simulink model "myGuyton_corrected_new"  (Simulink 6.6)
settings: Solver=ode15s  StartTime=0  StopTime=60*24*14  FixedStep=0.025  MaxStep=1  MinStep=0.00000001  RelTol=1e-1
values from neighbouring files (symbols this model uses):
  A1K = 0.5    [G92_var_decl_exp.m]
  A2K = 60    [G92_var_decl_exp.m]
  A3K = 40000    [G92_var_decl_exp.m]
  A4K = 0.1    [G92_var_decl_exp.m]
  A4K2 = 40000    [G92_var_decl_exp.m]
  AARK = 1    [G92_var_decl_exp.m]
  AARLL = 4    [G92_var_decl_exp.m]
  ADHC_IC = 1.01449    [G92_var_decl_exp.m]
  ADHINF = 0    [G92_var_decl_exp.m]
  ADHKLL = 0.2    [G92_var_decl_exp.m]
  ADHKUL = 5    [G92_var_decl_exp.m]
  ADHPAM = 0.3    [G92_var_decl_exp.m]
  ADHPUL = 85    [G92_var_decl_exp.m]
  ADHTC = 15    [G92_var_decl_exp.m]
  ADHVLL = 0.93617    [G92_var_decl_exp.m]
  ADHVUL = 2.5    [G92_var_decl_exp.m]
  AH10 = 0.333    [G92_var_decl_exp.m]
  AH11 = 1000    [G92_var_decl_exp.m]
  AH9 = 1    [G92_var_decl_exp.m]
  AHMNAR = 0.3    [G92_var_decl_exp.m]
  AHTHM = 2    [G92_var_decl_exp.m]
  AHY_IC = -0.461862    [G92_var_decl_exp.m]
  ALCLK = 0.3    [G92_var_decl_exp.m]
  ALDINF = 0    [G92_var_decl_exp.m]
  ALDKNS = 0    [G92_var_decl_exp.m]
  ALDMM = 2.5    [G92_var_decl_exp.m]
  AM1LL = 0    [G92_var_decl_exp.m]
  AM1UL = 5    [G92_var_decl_exp.m]
  AMC_IC = 1.05537    [G92_var_decl_exp.m]
  AMCSNS = 0.65    [G92_var_decl_exp.m]
  AMKM = 0.5    [G92_var_decl_exp.m]
  AMKMUL = 12    [G92_var_decl_exp.m]
  AMM1_IC = 1.00227    [G92_var_decl_exp.m]
  AMM2_IC = 1.09458    [G92_var_decl_exp.m]
  AMM4 = 0.005    [G92_var_decl_exp.m]
  AMNALL = 0.04    [G92_var_decl_exp.m]
  AMNAM = 0.8    [G92_var_decl_exp.m]
  AMNAUL = 15    [G92_var_decl_exp.m]
  AMT = 60    [G92_var_decl_exp.m]
  ANC_IC = 0.867681    [G92_var_decl_exp.m]
  ANCSNS = 0.4    [G92_var_decl_exp.m]
  ANGINF = 0    [G92_var_decl_exp.m]
  ANGKNS = 0    [G92_var_decl_exp.m]
  ANMALD = 2.5    [G92_var_decl_exp.m]
  ANMAM = 1.4    [G92_var_decl_exp.m]
  ANMARL = 0.86    [G92_var_decl_exp.m]
  ANMEM = 1.6    [G92_var_decl_exp.m]
  ANMKEL = 0.3    [G92_var_decl_exp.m]
  ANMKEM = 2    [G92_var_decl_exp.m]
  ANMLL = 0.7    [G92_var_decl_exp.m]
  ANMNAM = 1    [G92_var_decl_exp.m]
  ANMSLT = 2    [G92_var_decl_exp.m]
  ANMTM = 1.5    [G92_var_decl_exp.m]
  ANMUL = 1.8    [G92_var_decl_exp.m]
  ANPC_IC = 0.9333    [G92_var_decl_exp.m]
  ANPINF = 0    [G92_var_decl_exp.m]
  ANPKNS = 0    [G92_var_decl_exp.m]
  ANPTC = 4    [G92_var_decl_exp.m]
  ANPXAF = 1.5    [G92_var_decl_exp.m]
  ANPXUL = 10    [G92_var_decl_exp.m]
  ANT = 12    [G92_var_decl_exp.m]
  ANULL = 0.8    [G92_var_decl_exp.m]
  ANUM = 6    [G92_var_decl_exp.m]
  ANUVM = 0    [G92_var_decl_exp.m]
  ANV = 5000    [G92_var_decl_exp.m]
  ANX1_IC = 0    [G92_var_decl_exp.m]
  ANXM = 0    [G92_var_decl_exp.m]
  ANY = -0.2    [G92_var_decl_exp.m]
  AR1_IC = 1.00197    [G92_var_decl_exp.m]
  AR2_IC = 1.00306    [G92_var_decl_exp.m]
  AR3_IC = 1.05777    [G92_var_decl_exp.m]
  ARF = 0.5    [G92_var_decl_exp.m]
  ATRFBM = 0    [G92_var_decl_exp.m]
  ATRVM = 0    [G92_var_decl_exp.m]
  AU1_IC = 0.99999    [G92_var_decl_exp.m]
  AU4_IC = -0.00833091    [G92_var_decl_exp.m]
  AU6_IC = 1.00041    [G92_var_decl_exp.m]
  AUC1 = 0.3    [G92_var_decl_exp.m]
  AUDMP = 0.3    [G92_var_decl_exp.m]
  AUK = 0.004    [G92_var_decl_exp.m]
  AUL = 1.5    [G92_var_decl_exp.m]
  AULPM = 0    [G92_var_decl_exp.m]
  AUM1 = 3    [G92_var_decl_exp.m]
  AUM2 = 1    [G92_var_decl_exp.m]
  AUMAX = 5    [G92_var_decl_exp.m]
  AUMIN = 0.4    [G92_var_decl_exp.m]
  AUMK1 = 0.3    [G92_var_decl_exp.m]
  AUN1 = 0.5    [G92_var_decl_exp.m]
  AUS = 1    [G92_var_decl_exp.m]
  AUSLP = 1.5    [G92_var_decl_exp.m]
  AUTOGN = 7    [G92_var_decl_exp.m]
  AUTOK = 0.1    [G92_var_decl_exp.m]
  AUTOSN = 0.9    [G92_var_decl_exp.m]
  AUV = 0.55    [G92_var_decl_exp.m]
  AUX = 1    [G92_var_decl_exp.m]
  AUY = 0    [G92_var_decl_exp.m]
  BAROTC = 0.16    [G92_var_decl_exp.m]
  CFC = 0.01167    [G92_var_decl_exp.m]
  CKEEX = 4    [G92_var_decl_exp.m]
  CMPTSS = 2    [G92_var_decl_exp.m]
  CN2 = 0.0212    [G92_var_decl_exp.m]
  CN3_IC = 0.359907    [G92_var_decl_exp.m]
  CN7 = 0.2    [G92_var_decl_exp.m]
  CNR = 139    [G92_var_decl_exp.m]
  CPF = 0.0003    [G92_var_decl_exp.m]
  CPK = 0.000253    [G92_var_decl_exp.m]
  CPR = 40    [G92_var_decl_exp.m]
  CRRFLX = 0    [G92_var_decl_exp.m]
  CV = 0.1    [G92_var_decl_exp.m]
  DFP_IC = 1.16492e-06    [G92_var_decl_exp.m]
  DHDTR = 0.05    [G92_var_decl_exp.m]
  DIURET = 1    [G92_var_decl_exp.m]
  DR = 0    [G92_var_decl_exp.m]
  DTKA_IC = 0.0368507    [G92_var_decl_exp.m]
  DTNAR = 0.675    [G92_var_decl_exp.m]
  DTNARL = 1e-06    [G92_var_decl_exp.m]
  EARK = 1    [G92_var_decl_exp.m]
  EARLL = 24    [G92_var_decl_exp.m]
  EFAFR = 0    [G92_var_decl_exp.m]
  EXC = 1    [G92_var_decl_exp.m]
  ... (+137 more)
libraries: simulink x5
(part 3 of 3)

== system myGuyton_corrected_new/CIRCULATION/RPV Calculation ==
  PLA : Inport  Orientation=up
  CD5 : Product  Inputs=*/  OutScaling=2^-10
  Constant12 : Constant  Value=18
  Constant13 : Constant
  Gain13 : Gain  Gain=0.0357
  Sum18 : Sum  Inputs=|++
  RPV : Outport
  wires:
  Constant12/1 -> Sum18/1
  Sum18/1 -> Gain13/1  "PL1"
  Gain13/1 -> CD5/2
  Constant13/1 -> CD5/1
  PLA/1 -> Sum18/2
  CD5/1 -> RPV/1  "RPV"

== system myGuyton_corrected_new/CIRCULATION/RV1 Calculation ==
  PC : Inport  Orientation=left
  CD55 : Product  Orientation=left  Inputs=/*  OutScaling=2^-10
  Constant : Constant  Orientation=left  Value=17
  Constant1 : Constant  Orientation=left  Value=RVSM
  DAMPING : Subsystem  Orientation=left
      mask Display: dpoly([0 1],[1/0.1 1])
  Gain3 : Gain  Orientation=left  Gain=CN7
  Gain4 : Gain  Orientation=left  Gain=CN2
  Sum1 : Sum  Orientation=left  Inputs=-+|
  Sum2 : Sum  Orientation=left  Inputs=++|
  RV1 : Outport  Orientation=left
  wires:
  Constant/1 -> Sum1/1, Sum2/1
  Sum1/1 -> Gain3/1
  Gain3/1 -> Sum2/2
  Sum2/1 -> Gain4/1
  Gain4/1 -> DAMPING/1(In1)  "CN3"
  Constant1/1 -> CD55/2
  PC/1 -> Sum1/2
  CD55/1 -> RV1/1  "RV1"
  DAMPING/1(CN3) -> CD55/1

== system myGuyton_corrected_new/Capillary Dynamics, Tissue Fluid and Tissue Pprotein /CHY Calculation ==
  VTS : Inport
  60 : Product  Inputs=*/  OutScaling=2^-10
  Constant11 : Constant  Value=HYL
  Constant12 : Constant  Value=CMPTSS
  Gain8 : Gain  Gain=5
  POW3 : Math  Operator=pow  SaturateOnIntegerOverflow=on
  CHY : Outport
  wires:
  Constant11/1 -> 60/1
  Gain8/1 -> 60/2
  60/1 -> POW3/1
  Constant12/1 -> POW3/2
  VTS/1 -> Gain8/1
  POW3/1 -> CHY/1  "CHY"

== system myGuyton_corrected_new/Capillary Dynamics, Tissue Fluid and Tissue Pprotein /DLP Calculation ==
  CPP : Inport
  Constant5 : Constant  Value=CPR
  Constant6 : Constant  Value=LPDE
  Constant7 : Constant  Value=LPPR
  Gain6 : Gain  Gain=LPK
  Math Function2 : Math  Operator=pow  SaturateOnIntegerOverflow=on
  Saturation1 : Saturate  UpperLimit=inf  LowerLimit=0
  Sum6 : Sum  Inputs=+-|
  Sum7 : Sum  Inputs=|-+
  DLP : Outport
  wires:
  Constant6/1 -> Math Function2/2
  Math Function2/1 -> Gain6/1
  Gain6/1 -> Sum7/1
  Constant7/1 -> Sum7/2
  Sum7/1 -> DLP/1  "DLP"
  Saturation1/1 -> Math Function2/1  "CPPD"
  CPP/1 -> Sum6/1  "CPP"
  Constant5/1 -> Sum6/2
  Sum6/1 -> Saturation1/1

== system myGuyton_corrected_new/Capillary Dynamics, Tissue Fluid and Tissue Pprotein /FUN6 ==
  VTS : Inport
  FUN6 : simulink/Lookup Tables/Lookup Table (n-D)  numDimsPopupSelect=1  bp1=[0 12 15 18 21 24]  bp2=[10,22,31]  bp3=[1:3]  bp4=[1:3]  bpcell={ [1:3], [1:3] }  explicitNumDims=2  searchMode=Binary Search  cacheBpFlag=off  vectorInputFlag=off  tableData=[0 11.4 14 16 17.3 18]  interpMethod=Cubic Spline  extrapMethod=None - Clip  rangeErrorMode=None
  VG : Outport
  wires:
  VTS/1 -> FUN6/1
  FUN6/1 -> VG/1  "VG"

== system myGuyton_corrected_new/Capillary Dynamics, Tissue Fluid and Tissue Pprotein /PPC Calculation ==
  CPP : Inport  Orientation=left
  Constant4 : Constant  Orientation=left  Value=2
  Gain3 : Gain  Orientation=left  Gain=0.28
  Gain4 : Gain  Orientation=left  Gain=0.0019
  Math Function1 : Math  Orientation=left  Operator=pow  SaturateOnIntegerOverflow=on
  Sum4 : Sum  Orientation=left  Inputs=|++
  PPC : Outport  Orientation=left
  wires:
  Constant4/1 -> Math Function1/2
  Math Function1/1 -> Gain4/1
  Gain4/1 -> Sum4/2
  Gain3/1 -> Sum4/1
  CPP/1 -> Math Function1/1, Gain3/1  "CPP"
  Sum4/1 -> PPC/1  "PPC"

== system myGuyton_corrected_new/Capillary Dynamics, Tissue Fluid and Tissue Pprotein /PTCRP Calculation ==
  CPI : Inport  Orientation=down
  Constant13 : Constant  Value=2
  Gain10 : Gain  Gain=0.0019
  Gain9 : Gain  Gain=0.28
  POW1 : Math  Operator=pow  SaturateOnIntegerOverflow=on
  Sum14 : Sum  Inputs=++|
  PTCRP : Outport
  wires:
  Constant13/1 -> POW1/2
  POW1/1 -> Gain10/1
  Gain10/1 -> Sum14/1
  Gain9/1 -> Sum14/2
  CPI/1 -> Gain9/1, POW1/1
  Sum14/1 -> PTCRP/1  "PTCPR"

== system myGuyton_corrected_new/Capillary Dynamics, Tissue Fluid and Tissue Pprotein /PTT Calculation ==
  VTS1 : Inport
  1 : Product  Inputs=*/  OutScaling=2^-10
  Constant15 : Constant  Value=VTSF
  Constant16 : Constant  Value=2
  POW2 : Math  Operator=pow  SaturateOnIntegerOverflow=on
  Sum17 : Sum  Inputs=|+-
  PTT : Outport
  wires:
  Constant15/1 -> Sum17/2, 1/2  "VTSF"
  Sum17/1 -> 1/1
  1/1 -> POW2/1
  Constant16/1 -> POW2/2
  VTS1/1 -> Sum17/1
  POW2/1 -> PTT/1  "PTT"

== system myGuyton_corrected_new/Capillary Dynamics, Tissue Fluid and Tissue Pprotein /VTCPL Calculation ==
  PC : Inport  Orientation=down
  Constant : Constant  Value=PCR
  Constant1 : Constant  Value=PCE
  Gain1 : Gain  Gain=CPK
  Math Function : Math  Operator=pow  SaturateOnIntegerOverflow=on
  Saturation : Saturate  UpperLimit=inf  LowerLimit=0
  Sum1 : Sum  Inputs=+-|
  VTCPL : Outport
  wires:
  Constant/1 -> Sum1/2
  Sum1/1 -> Saturation/1  "PRCD"
  Saturation/1 -> Gain1/1
  Gain1/1 -> Math Function/1
  Constant1/1 -> Math Function/2
  PC/1 -> Sum1/1
  Math Function/1 -> VTCPL/1  "VTCPL"

== system myGuyton_corrected_new/Capillary Dynamics, Tissue Fluid and Tissue Pprotein /VTS1 Calculation ==
  VTS : Inport
  Constant : Constant  Value=12
  Gain : Gain  Gain=TSSLML
  Sum : Sum  Inputs=|+-
  Sum2 : Sum  Inputs=|-+
  VTS2 TF : Subsystem
      mask Display: dpoly([0 1], [1/TSSLTC 1] )
  VTS1 : Outport
  wires:
  VTS/1 -> Sum/1, Sum2/2  "VTS"
  Constant/1 -> Sum/2
  Sum/1 -> Gain/1
  Gain/1 -> VTS2 TF/1(In1)
  Sum2/1 -> VTS1/1
  VTS2 TF/1(VTS2) -> Sum2/1  "VTS2"

== system myGuyton_corrected_new/Heart Hypertrophy or Deteoration/Hypertr. Eff. on LV ==
  In1 : Inport
  HH4 : Gain  Gain=1/57600
  HH5 : Integrator  InitialConditionSource=external
  IC_HPL : Constant  Value=HPL_IC
  Sum1 : Sum  Inputs=|+-
  HPL : Outport
  wires:
  Sum1/1 -> HH4/1
  HH4/1 -> HH5/1
  HH5/1 -> Sum1/2, HPL/1
  IC_HPL/1 -> HH5/2
  In1/1 -> Sum1/1

== system myGuyton_corrected_new/Heart Hypertrophy or Deteoration/Hypertr. Eff. on RV ==
  In1 : Inport
  HH10 : Integrator  InitialConditionSource=external
  HH9 : Gain  Gain=1/57600
  IC_HPR : Constant  Value=HPR_IC
  Sum1 : Sum  Inputs=|+-
  HPR : Outport
  wires:
  Sum1/1 -> HH9/1
  HH9/1 -> HH10/1
  HH10/1 -> Sum1/2, HPR/1
  IC_HPR/1 -> HH10/2
  In1/1 -> Sum1/1

== system myGuyton_corrected_new/KIDNEYS/AAR Calculation ==
  AAR1 : Inport
  ANPX : Inport  Port=2
  ANMARL2 : Saturate  UpperLimit=inf  LowerLimit=AARLL
  Constant6 : Constant  Value=ANPXAF
  Product3 : Product  RndMeth=Zero
  Sum10 : Sum  Inputs=|++
  Sum9 : Sum  Inputs=|-+
  AAR : Outport
  wires:
  ANPX/1 -> Product3/1
  Constant6/1 -> Product3/2, Sum9/2
  Product3/1 -> Sum9/1
  Sum9/1 -> Sum10/2
  Sum10/1 -> ANMARL2/1  "AAR"
  ANMARL2/1 -> AAR/1  "AAR"
  AAR1/1 -> Sum10/1

== system myGuyton_corrected_new/KIDNEYS/ANMAR/ANMER Calculation ==
  ANM : Inport
  ANMARL : Saturate  UpperLimit=inf  LowerLimit=ANMARL
  Constant1 : Constant
  Gain2 : Gain  Gain=ANMEM
  Gain3 : Gain  Gain=ANMAM
  Sum2 : Sum  Inputs=|+-
  Sum3 : Sum  Inputs=|++
  Sum4 : Sum  Inputs=-+|
  Sum5 : Sum  Inputs=++|
  ANMER : Outport
  ANMAR : Outport  Port=2
  wires:
  ANM/1 -> Sum2/1, Sum4/2
  Constant1/1 -> Sum2/2, Sum3/2, Sum5/1, Sum4/1  "1"
  Sum2/1 -> Gain2/1
  Gain2/1 -> Sum3/1
  Sum4/1 -> Gain3/1
  Gain3/1 -> Sum5/2
  Sum5/1 -> ANMARL/1  "ANMAR"
  Sum3/1 -> ANMER/1  "ANMER"
  ANMARL/1 -> ANMAR/1  "ANMAR"

== system myGuyton_corrected_new/KIDNEYS/ANMKE Calculation ==
  ANM : Inport  Orientation=left
  Constant10 : Constant  Orientation=left
  Gain14 : Gain  Orientation=left  Gain=ANMKEM
  Saturation : Saturate  Orientation=left  UpperLimit=inf  LowerLimit=ANMKEL
  Sum : Sum  Orientation=left  Inputs=|+-
  Sum15 : Sum  Orientation=left  Inputs=|++
  ANMKE : Outport  Orientation=left
  wires:
  Constant10/1 -> Sum/2, Sum15/2
  Sum/1 -> Gain14/1
  Gain14/1 -> Sum15/1
  ANM/1 -> Sum/1
  Sum15/1 -> Saturation/1  "ANMKE"
  Saturation/1 -> ANMKE/1

== system myGuyton_corrected_new/KIDNEYS/AUMK Calculation ==
  AUM : Inport
  Constant : Constant
  Gain1 : Gain  Gain=ARF
  Saturation : Saturate  UpperLimit=inf  LowerLimit=0.8
  Sum : Sum  Inputs=|+-
  Sum1 : Sum  Inputs=|++
  AUMK : Outport
  wires:
  Constant/1 -> Sum/2, Sum1/2
  Sum/1 -> Gain1/1
  Gain1/1 -> Sum1/1
  Sum1/1 -> Saturation/1  "AUMK"
  Saturation/1 -> AUMK/1  "AUMK"
  AUM/1 -> Sum/1

== system myGuyton_corrected_new/KIDNEYS/AUMKT Calculation ==
  AUMK : Inport
  Constant : Constant
  Gain2 : Gain  Gain=AUMK1
  Sum12 : Sum  Inputs=|+-
  Sum2 : Sum  Inputs=|++
  AUMKT : Outport
  wires:
  Constant/1 -> Sum12/2, Sum2/2
  Sum12/1 -> Gain2/1
  Gain2/1 -> Sum2/1
  Sum2/1 -> AUMKT/1  "AUMKT"
  AUMK/1 -> Sum12/1

== system myGuyton_corrected_new/KIDNEYS/DTKA Dynamics ==
  In1 : Inport
  Constant8 : Constant  Value=DTKA_IC
  Gain14 : Gain  Gain=I6
  Integrator : Integrator  InitialConditionSource=external
  Sum15 : Sum  Inputs=-+|
  DTKA : Outport
  wires:
  Sum15/1 -> Gain14/1
  Gain14/1 -> Integrator/1
  Constant8/1 -> Integrator/2
  Integrator/1 -> Sum15/1, DTKA/1  "DTKA"
  In1/1 -> Sum15/2

== system myGuyton_corrected_new/KIDNEYS/DTNANG Calculation ==
  ANM : Inport
  ANMARL6 : Saturate  UpperLimit=inf  LowerLimit=0
  Constant10 : Constant
  Gain14 : Gain  Gain=ANMNAM
  Gain17 : Gain  Gain=0.1
  Sum : Sum  Inputs=|+-
  Sum15 : Sum  Inputs=|++
  DTNANG : Outport
  wires:
  Constant10/1 -> Sum/2, Sum15/2
  Sum/1 -> Gain14/1
  Gain14/1 -> Sum15/1
  Sum15/1 -> Gain17/1
  Gain17/1 -> ANMARL6/1
  ANM/1 -> Sum/1
  ANMARL6/1 -> DTNANG/1  "DTNANG"

== system myGuyton_corrected_new/KIDNEYS/DTURI/UROD Calculation ==
  GFN : Inport  Orientation=down
  VTW : Inport  Port=2
  Constant8 : Constant  Value=URFORM
  Divide4 : Product  Inputs=*/  OutScaling=2^-10
  Gain14 : Gain  Gain=3.84
  Gain15 : Gain  Orientation=left  Gain=REK
  Integrator : Integrator  InitialConditionSource=external
  PLUR_IC : Constant  Value=PLUR_IC
  Product5 : Product  Inputs=3  RndMeth=Zero
  Sum15 : Sum  Inputs=|+-
  DTURI : Outport
  wires:
  Gain14/1 -> Gain15/1, DTURI/1  "DTURI"
  Divide4/1 -> Product5/3  "PLURC"
  Product5/1 -> Gain14/1
  Gain15/1 -> Sum15/2  "UROD"
  Constant8/1 -> Sum15/1  "URFORM"
  Sum15/1 -> Integrator/1
  PLUR_IC/1 -> Integrator/2
  Integrator/1 -> Divide4/1  "PLUR"
  VTW/1 -> Divide4/2
  GFN/1 -> Product5/1, Product5/2

== system myGuyton_corrected_new/KIDNEYS/GFN DAMPING ==
  In1 : Inport
  Constant2 : Constant  Value=GFN_IC
  Gain3 : Gain  Gain=1/9
  Integrator : Integrator  InitialConditionSource=external
  Sum5 : Sum  Inputs=|+-
  GFN : Outport
  wires:
  Sum5/1 -> Gain3/1
  In1/1 -> Sum5/1
  Integrator/1 -> Sum5/2, GFN/1  "GFN"
  Gain3/1 -> Integrator/1
  Constant2/1 -> Integrator/2

== system myGuyton_corrected_new/KIDNEYS/GLPC Calculation ==
  VP : Inport
  RFN : Inport  Port=2
  VB : Inport  Port=3
  GFN : Inport  Port=4
  PPC : Inport  Port=5
  Constant11 : Constant  Value=4
  Constant12 : Constant  Value=1.35
  Constant3 : Constant  Value=GLPCA
  EFAFPR CALCULATION : Subsystem
  Gain14 : Gain  Gain=0.98
  IF GLPCA>0 : Switch  Criteria=u2 > Threshold
  Math Function1 : Math  Operator=pow  SaturateOnIntegerOverflow=on
  Product7 : Product  RndMeth=Zero
  Subsystem : Subsystem
      mask Display: dpoly([0 1],[GPPD 1])
  Sum1 : Sum  Inputs=|++
  GLPC : Outport
  wires:
  EFAFPR CALCULATION/1(EFAFPR) -> Math Function1/1  "EFAFPR"
  Constant3/1 -> IF GLPCA>0/2
  PPC/1 -> Sum1/1, Product7/2
  Constant11/1 -> Sum1/2
  Sum1/1 -> IF GLPCA>0/3  "PPC+4"
  Constant12/1 -> Math Function1/2
  Math Function1/1 -> Product7/1
  Product7/1 -> Gain14/1
  RFN/1 -> EFAFPR CALCULATION/2(RFN)
  GFN/1 -> EFAFPR CALCULATION/4(GFN)
  VP/1 -> EFAFPR CALCULATION/1(VP)
  VB/1 -> EFAFPR CALCULATION/3(VB)
  IF GLPCA>0/1 -> GLPC/1  "GLPC"
  Gain14/1 -> Subsystem/1(In1)  "GLPC"
  Subsystem/1(Out1) -> IF GLPCA>0/1

== system myGuyton_corrected_new/KIDNEYS/MDFLK Calculation ==
  MDFLW : Inport  Orientation=left
  ANMARL6 : Saturate  Orientation=left  UpperLimit=inf  LowerLimit=0.1
  Constant10 : Constant
  Gain14 : Gain  Orientation=left  Gain=MDFLKM
  Sum15 : Sum  Orientation=left  Inputs=|+-
  Sum18 : Sum  Orientation=left  Inputs=|++
  MDFLK : Outport  Orientation=left
  wires:
  Constant10/1 -> Sum15/2, Sum18/2
  Sum15/1 -> Gain14/1
  Gain14/1 -> Sum18/1
  Sum18/1 -> ANMARL6/1
  MDFLW/1 -> Sum15/1
  ANMARL6/1 -> MDFLK/1  "MDFLK"

== system myGuyton_corrected_new/KIDNEYS/MDFLW Calculation ==
  GFN : Inport
  ANMARL3 : Saturate  UpperLimit=inf  LowerLimit=0
  Constant6 : Constant
  Gain7 : Gain  Gain=8
  Gain8 : Gain  Gain=MDFL1
  Sum5 : Sum  Inputs=-+|
  Sum9 : Sum  Inputs=++|
  MDFLW : Outport
  wires:
  Gain7/1 -> Sum5/2  "PTFL"
  Constant6/1 -> Sum5/1, Sum9/1
  Sum5/1 -> Gain8/1
  Gain8/1 -> Sum9/2
  Sum9/1 -> ANMARL3/1  "MDFLW"
  GFN/1 -> Gain7/1
  ANMARL3/1 -> MDFLW/1  "MDFLW"

== system myGuyton_corrected_new/KIDNEYS/PAR Calculation ==
  PA : Inport
  Constant : Constant  Value=GBL
  Constant1 : Constant  Value=RAPRSP
  Constant2 : Constant  Value=RFCDFT
  Constant3 : Constant  Value=100
  Gain : Gain  Gain=RCDFPC
  PAR TF : Subsystem
      mask Display: dpoly([0 1],[RCDFDP 1])
  Sum : Sum  Inputs=|+-
  Sum1 : Sum  Inputs=|+-
  Sum2 : Sum  Inputs=|++
  Switch : Switch  Criteria=u2 > Threshold
  Switch1 : Switch  Criteria=u2 > Threshold
  PAR : Outport
  wires:
  PA/1 -> Sum/1, Sum1/1
  Constant/1 -> Sum/2
  Sum/1 -> Switch/3  "PAR"
  Constant1/1 -> Switch/2, Switch/1
  Switch/1 -> Switch1/3  "PAR"
  Constant2/1 -> Switch1/2
  Constant3/1 -> Sum1/2, Sum2/2
  Sum1/1 -> Sum2/1  "PA-100"
  Sum2/1 -> Gain/1
  Gain/1 -> PAR TF/1(In1)
  PAR TF/1(PAR) -> Switch1/1  "PAR"
  Switch1/1 -> PAR/1  "PAR"

== system myGuyton_corrected_new/KIDNEYS/RCPRS Calculation ==
  RFN : Inport
  Constant2 : Constant  Value=1.2
  Gain1 : Gain  Gain=RFABX
  Gain4 : Gain  Gain=RVRS
  Sum1 : Sum  Inputs=|+-
  Sum7 : Sum  Inputs=|++
  RCPRS : Outport
  wires:
  Constant2/1 -> Sum1/2, Sum7/2
  Sum1/1 -> Gain1/1
  Gain1/1 -> Sum7/1
  Sum7/1 -> Gain4/1
  RFN/1 -> Sum1/1
  Gain4/1 -> RCPRS/1  "RCPRS"

== system myGuyton_corrected_new/KIDNEYS/RFABD Calculation ==
  RABSPR : Inport
  ANMARL2 : Saturate  UpperLimit=inf  LowerLimit=0.0001
  Constant5 : Constant
  DAMPING : Subsystem
      mask Display: dpoly([0 1],[RFABDP 1])
  Gain4 : Gain  Gain=RABSC
  Gain5 : Gain  Gain=RFABDM
  Sum10 : Sum  Inputs=|++
  Sum9 : Sum  Inputs=|+-
  RFABD : Outport
  wires:
  Gain4/1 -> DAMPING/1(RFAB1)  "RFAB"
  Constant5/1 -> Sum9/2, Sum10/2
  Sum9/1 -> Gain5/1
  Gain5/1 -> Sum10/1
  Sum10/1 -> ANMARL2/1
  ANMARL2/1 -> RFABD/1  "RFABD"
  RABSPR/1 -> Gain4/1
  DAMPING/1(RFAB) -> Sum9/1

== system myGuyton_corrected_new/KIDNEYS/RNAUG1 Calculation ==
  MDFLW : Inport
  ANMARL3 : Saturate  Orientation=left  UpperLimit=RNAUUL  LowerLimit=RNAULL
  Constant6 : Constant  Orientation=left
  Constant7 : Constant  Orientation=left
  Gain7 : Gain  Orientation=left  Gain=RNAUGN
  Subsystem5 : Subsystem  Orientation=left
      mask Display: dpoly([0 1],[RNAGTC 1])
  Sum5 : Sum  Orientation=down  Inputs=+-
  Sum9 : Sum  Orientation=left  Inputs=|++
  RNAUG1 : Outport  Orientation=left
  wires:
  Constant6/1 -> Sum5/2
  Sum5/1 -> Gain7/1
  Gain7/1 -> Sum9/1
  Constant7/1 -> Sum9/2
  Sum9/1 -> Subsystem5/1(In1)
  Subsystem5/1(RNAUG1) -> ANMARL3/1
  MDFLW/1 -> Sum5/1
  ANMARL3/1 -> RNAUG1/1  "RNAUG1"

== system myGuyton_corrected_new/KIDNEYS/RNAUG2 Calculation ==
  RNAUG1 : Inport  Orientation=left
  Constant6 : Constant
  Constant7 : Constant  Value=RNAUG3_IC
  Gain7 : Gain  Gain=RNAUAD
  Integrator : Integrator  InitialConditionSource=external
  Sum : Sum  Orientation=left  Inputs=|+-
  Sum5 : Sum  Inputs=|+-
  RNAUG2 : Outport  Orientation=left
  wires:
  Sum/1 -> Sum5/1, RNAUG2/1  "RNAUG2"
  Integrator/1 -> Sum/2  "RNAUG3"
  Constant6/1 -> Sum5/2
  Sum5/1 -> Gain7/1
  Gain7/1 -> Integrator/1
  Constant7/1 -> Integrator/2
  RNAUG1/1 -> Sum/1

== system myGuyton_corrected_new/KIDNEYS/RNAUG2T Calculation ==
  RNAUG2 : Inport  Orientation=left
  Constant1 : Constant  Orientation=left
  Gain2 : Gain  Orientation=left  Gain=EFAFR
  Sum : Sum  Orientation=left  Inputs=|+-
  Sum2 : Sum  Orientation=left  Inputs=|++
  RNAUG2T : Outport  Orientation=left
  wires:
  Constant1/1 -> Sum/2, Sum2/2
  Sum/1 -> Gain2/1
  Gain2/1 -> Sum2/1
  RNAUG2/1 -> Sum/1
  Sum2/1 -> RNAUG2T/1

== system myGuyton_corrected_new/Muscle O2 Delivery/Damping Z6 ==
  OVS1 : Inport
  Constant : Constant  Value=OVS_IC
  Gain1 : Gain  Gain=1/60
  Integrator : Integrator  InitialConditionSource=external
  Sum1 : Sum  Inputs=|+-
  OVS : Outport
  wires:
  OVS1/1 -> Sum1/1
  Integrator/1 -> OVS/1, Sum1/2
  Gain1/1 -> Integrator/1
  Sum1/1 -> Gain1/1
  Constant/1 -> Integrator/2

== system myGuyton_corrected_new/Non-muscle O2 Delivery/Damping Z7 ==
  In1 : Inport
  CONSTANT1 : Constant  Value=OSV_IC
  Gain1 : Gain  Gain=1/15
  Integrator : Integrator  InitialConditionSource=external
  Sum1 : Sum  Inputs=|+-
  OSV : Outport
  wires:
  Sum1/1 -> Gain1/1
  Gain1/1 -> Integrator/1
  Integrator/1 -> Sum1/2, OSV/1
  In1/1 -> Sum1/1
  CONSTANT1/1 -> Integrator/2

== system myGuyton_corrected_new/Pulmonary Fluid Dynamics/Damping Z18 ==
  PPZ : Inport
  Gain1 : Gain  Gain=1/15
  Integrator : Integrator  InitialConditionSource=external
  PPD_IC : Constant  Value=PPD_IC
  Sum1 : Sum  Inputs=|+-
  PPD : Outport
  wires:
  Sum1/1 -> Gain1/1
  Gain1/1 -> Integrator/1
  Integrator/1 -> Sum1/2, PPD/1
  PPZ/1 -> Sum1/1
  PPD_IC/1 -> Integrator/2

== system myGuyton_corrected_new/Pulmonary Fluid Dynamics/Damping Z19 ==
  DFZ : Inport
  Gain1 : Gain  Gain=1/15
  Integrator : Integrator  InitialConditionSource=external
  PPD_IC : Constant  Value=DFP_IC
  Sum1 : Sum  Inputs=|+-
  DFP : Outport
  wires:
  PPD_IC/1 -> Integrator/2
  DFZ/1 -> Sum1/1
  Integrator/1 -> DFP/1, Sum1/2
  Gain1/1 -> Integrator/1
  Sum1/1 -> Gain1/1

== system myGuyton_corrected_new/Pulmonary Oxygen Uptake/O2VAD2 Calculation ==
  PO2ART : Inport  Orientation=left
  Constant4 : Constant  Orientation=left  Value=67
  Constant5 : Constant  Value=30
  Constant6 : Constant  Orientation=left
  Constant7 : Constant
  Constant8 : Constant
  Divide3 : Product  Orientation=left  Inputs=*/  OutScaling=2^-10
  Divide4 : Product  Orientation=left  Inputs=*/  OutScaling=2^-10
  Gain3 : Gain  Orientation=left  Gain=3
  O2VAD1 DYNAMICS : Subsystem  Orientation=left
      mask Display: dpoly([0 1],[1/0.0005 1])
  Saturation : Saturate  Orientation=left  UpperLimit=1  LowerLimit=0.6
  Sum5 : Sum  Orientation=left  Inputs=|+-
  Sum6 : Sum  Orientation=left  Inputs=|+-
  Sum7 : Sum  Inputs=|++
  O2VAD2 : Outport
  O2VTS2 : Outport  Port=2
  wires:
  Constant4/1 -> Sum5/2
  Sum5/1 -> Divide3/1
  Constant5/1 -> Divide3/2
  Divide3/1 -> Saturation/1  "O2VTST"
  Saturation/1 -> Divide4/2
  Constant6/1 -> Divide4/1
  Divide4/1 -> Sum6/1, O2VTS2/1  "O2VTS2"
  Constant7/1 -> Sum6/2
  Sum6/1 -> Gain3/1
  Gain3/1 -> O2VAD1 DYNAMICS/1(In1)
  O2VAD1 DYNAMICS/1(O2VAD1) -> Sum7/2  "O2VAD1"
  Constant8/1 -> Sum7/1
  PO2ART/1 -> Sum5/1
  Sum7/1 -> O2VAD2/1  "O2VAD2"

== system myGuyton_corrected_new/Pulmonary Oxygen Uptake/PO2ART Calculation ==
  note: PO2/PO3/PO4
  OSA : Inport
  Constant : Constant  Value=46
  Constant1 : Constant  Value=0.8
  Constant2 : Constant  Value=74
  Constant3 : Constant  Value=0.936
  Constant4 : Constant  Value=114
  Constant5 : Constant
  Gain : Gain  Gain=205.882
  Gain1 : Gain  Gain=57.5
  Gain2 : Gain  Gain=625
  Gain3 : Gain  Gain=6667
  Sum : Sum  Inputs=|-+
  Sum1 : Sum  Inputs=|++
  Sum2 : Sum  Inputs=|-+
  Sum3 : Sum  Inputs=|++
  Sum4 : Sum  Inputs=|-+
  Sum5 : Sum  Inputs=|++
  Switch : Switch  Criteria=u2 > Threshold  Threshold=0.8
  Switch1 : Switch  Criteria=u2 > Threshold  Threshold=0.936
  Switch2 : Switch  Criteria=u2 > Threshold  Threshold=1
  PO2ART : Outport
  wires:
  OSA/1 -> Switch/2, Gain1/1, Sum/2, Sum2/2, Switch1/2, Sum4/2, Switch2/2  "OSA"
  Switch/1 -> Switch1/3  "PO3/PO4"
  Constant1/1 -> Sum/1
  Constant/1 -> Sum1/1
  Sum/1 -> Gain/1
  Gain/1 -> Sum1/2
  Sum1/1 -> Switch/1  "PO3"
  Gain1/1 -> Switch/3  "PO4"
  Constant3/1 -> Sum2/1
  Sum2/1 -> Gain2/1
  Gain2/1 -> Sum3/2
  Constant2/1 -> Sum3/1
  Sum3/1 -> Switch1/1  "PO2"
  Switch1/1 -> Switch2/3
  Constant5/1 -> Sum4/1
  Sum4/1 -> Gain3/1
  Gain3/1 -> Sum5/2
  Constant4/1 -> Sum5/1
  Sum5/1 -> Switch2/1  "PO1"
  Switch2/1 -> PO2ART/1

== system myGuyton_corrected_new/Thirst, Drinking snd Salt Apetite/AHTH Calculation ==
  ADHC : Inport
  STH : Inport  Port=2
  0.001 : Gain  Gain=0.001
  13 : Saturate  UpperLimit=inf  LowerLimit=0
  8 : Product  RndMeth=Zero
  Constant5 : Constant
  Gain1 : Gain  Gain=AHTHM
  Sum3 : Sum  Inputs=|+-
  Sum4 : Sum  Inputs=|++
  AHTH : Outport
  wires:
  Constant5/1 -> Sum3/2, Sum4/2
  Sum3/1 -> Gain1/1
  Gain1/1 -> Sum4/1
  Sum4/1 -> 8/2
  8/1 -> 0.001/1
  STH/1 -> 8/1
  13/1 -> AHTH/1  "AHTH"
  ADHC/1 -> Sum3/1
  0.001/1 -> 13/1

== system myGuyton_corrected_new/Thirst, Drinking snd Salt Apetite/ANMTH Calculation ==
  ANM : Inport
  Constant1 : Constant
  Gain2 : Gain  Gain=ANMTM
  Gain3 : Gain  Gain=0.001
  Sum1 : Sum  Inputs=|+-
  ANMTH : Outport
  wires:
  Gain2/1 -> Gain3/1
  Constant1/1 -> Sum1/2
  Sum1/1 -> Gain2/1
  ANM/1 -> Sum1/1
  Gain3/1 -> ANMTH/1  "ANMTH"

== system myGuyton_corrected_new/Thirst, Drinking snd Salt Apetite/STH Calculation ==
  POT : Inport
  ANM : Inport  Port=2
  1A : Math  Operator=pow  SaturateOnIntegerOverflow=on
  2C : Product  Inputs=3  RndMeth=Zero
  3,4 : Saturate  UpperLimit=8  LowerLimit=0.8  LinearizeAsGain=off
  Constant : Constant  Value=Z10
  Constant1 : Constant  Value=2
  Constant2 : Constant  Value=Z11
  Constant3 : Constant
  Constant4 : Constant
  Gain : Gain  Gain=ANMSLT
  Sum : Sum  Inputs=|-+
  Sum1 : Sum  Inputs=|-+
  Sum2 : Sum  Inputs=|++
  STH : Outport
  wires:
  Constant/1 -> Sum/2
  Constant1/1 -> 1A/2
  Sum/1 -> 1A/1
  Constant3/1 -> Sum1/1
  Sum1/1 -> Gain/1
  Gain/1 -> Sum2/1
  Constant4/1 -> Sum2/2
  1A/1 -> 2C/1
  Constant2/1 -> 2C/2
  Sum2/1 -> 2C/3  "ANMSML"
  2C/1 -> 3,4/1
  POT/1 -> Sum/1
  3,4/1 -> STH/1
  ANM/1 -> Sum1/2

== system myGuyton_corrected_new/Thirst, Drinking snd Salt Apetite/TVDDynamics ==
  TVZ+DR : Inport
  16 : Integrator  InitialConditionSource=external
  ARN16 : Gain  Gain=1/TVDDL
  IC_TVD : Constant  Value=TVD_IC
  Sum6 : Sum  Inputs=|+-
  TVD : Outport
  wires:
  Sum6/1 -> ARN16/1
  ARN16/1 -> 16/1
  IC_TVD/1 -> 16/2
  16/1 -> Sum6/2, TVD/1  "TVD"
  TVZ+DR/1 -> Sum6/1

== system myGuyton_corrected_new/Vascular Stress Relaxation/VSR Long Term ==
  In1 : Inport
  IC_VV6 : Constant  Value=VV6_IC
  SR4A : Gain  Gain=1/SRK2
  SR5A : Integrator  InitialConditionSource=external
  Sum2 : Sum  Inputs=|+-
  VV6 : Outport
  wires:
  IC_VV6/1 -> SR5A/2
  SR5A/1 -> Sum2/2, VV6/1
  SR4A/1 -> SR5A/1
  Sum2/1 -> SR4A/1
  In1/1 -> Sum2/1

== system myGuyton_corrected_new/Vascular Stress Relaxation/VSR Short Term ==
  In1 : Inport
  IC_VV7 : Constant  Value=VV7_IC
  SR4 : Gain  Gain=1/SRK
  SR5 : Integrator  InitialConditionSource=external
  Sum3 : Sum  Inputs=|+-
  VV7 : Outport
  wires:
  Sum3/1 -> SR4/1
  SR4/1 -> SR5/1
  SR5/1 -> Sum3/2, VV7/1
  IC_VV7/1 -> SR5/2
  In1/1 -> Sum3/1

== system myGuyton_corrected_new/Volume Receptors/Volume Receptor Adaptation ==
  AHZ_a : Inport
  IC_AHY : Constant  Value=AHY_IC
  Integrator : Integrator  InitialConditionSource=external
  Sum : Sum  Inputs=|+-
  VR4 : Gain  Gain=1/AH11
  AHY : Outport  Orientation=up
  wires:
  Sum/1 -> VR4/1
  VR4/1 -> Integrator/1
  IC_AHY/1 -> Integrator/2
  Integrator/1 -> Sum/2, AHY/1
  AHZ_a/1 -> Sum/1

== system myGuyton_corrected_new/Autonomic Control of the Circulation/AUC3, AUN, AUC6/AUB ==
  PA1 : Inport
  AUC1_a2 : Constant  Value=160
  AUC_a : Constant  Value=0
  AUC_a1 : Constant  Value=1.3336
  Gain : Gain  Gain=0.016667
  Sum1 : Sum  Inputs=-+|
  "if PA1>=40, AUC = AUC If PA1 < 40, AUC = 0.02" : Switch  Threshold=80
  "if PA1>=80, AUC1 = 0 If PA1 < 80, AUC = 0.005 * (80-PA1);" : Switch  Threshold=160
  AUB : Outport
  wires:
  "if PA1>=80, AUC1 = 0 If PA1 < 80, AUC = 0.005 * (80-PA1);"/1 -> "if PA1>=40, AUC = AUC If PA1 < 40, AUC = 0.02"/1  "AUB"
  PA1/1 -> "if PA1>=80, AUC1 = 0 If PA1 < 80, AUC = 0.005 * (80-PA1);"/2, Sum1/1, "if PA1>=40, AUC = AUC If PA1 < 40, AUC = 0.02"/2  "PA1"
  "if PA1>=40, AUC = AUC If PA1 < 40, AUC = 0.02"/1 -> AUB/1  "AUB"
  AUC_a1/1 -> "if PA1>=40, AUC = AUC If PA1 < 40, AUC = 0.02"/3
  Gain/1 -> "if PA1>=80, AUC1 = 0 If PA1 < 80, AUC = 0.005 * (80-PA1);"/3
  Sum1/1 -> Gain/1
  AUC1_a2/1 -> Sum1/2
  AUC_a/1 -> "if PA1>=80, AUC1 = 0 If PA1 < 80, AUC = 0.005 * (80-PA1);"/1

== system myGuyton_corrected_new/Autonomic Control of the Circulation/AUC3, AUN, AUC6/AUC ==
  PA1 : Inport  Orientation=down
  AUC1 : Gain  Gain=AUC1
  AUC1_a2 : Constant  Value=80
  AUC_a : Constant  Value=0
  AUC_a1 : Constant  Value=0.2
  Gain : Gain  Gain=0.005
  Sum1 : Sum  Inputs=-+|
  "if PA1>=40, AUC = AUC If PA1 < 40, AUC = 0.02" : Switch  Threshold=40
  "if PA1>=80, AUC1 = 0 If PA1 < 80, AUC = 0.005 * (80-PA1);" : Switch  Threshold=80
  AUC : Outport
  wires:
  AUC_a/1 -> "if PA1>=80, AUC1 = 0 If PA1 < 80, AUC = 0.005 * (80-PA1);"/1
  AUC1_a2/1 -> Sum1/2
  Sum1/1 -> Gain/1
  Gain/1 -> "if PA1>=80, AUC1 = 0 If PA1 < 80, AUC = 0.005 * (80-PA1);"/3
  AUC_a1/1 -> "if PA1>=40, AUC = AUC If PA1 < 40, AUC = 0.02"/3
  "if PA1>=40, AUC = AUC If PA1 < 40, AUC = 0.02"/1 -> AUC1/1
  PA1/1 -> "if PA1>=40, AUC = AUC If PA1 < 40, AUC = 0.02"/2, Sum1/1, "if PA1>=80, AUC1 = 0 If PA1 < 80, AUC = 0.005 * (80-PA1);"/2
  "if PA1>=80, AUC1 = 0 If PA1 < 80, AUC = 0.005 * (80-PA1);"/1 -> "if PA1>=40, AUC = AUC If PA1 < 40, AUC = 0.02"/1  "AUC"
  AUC1/1 -> AUC/1  "AUC"

== system myGuyton_corrected_new/Autonomic Control of the Circulation/AUC3, AUN, AUC6/AUC2 ==
  PO2ART : Inport  Orientation=down
  AUC1_a2 : Constant  Value=80
  AUC_a : Constant  Value=0
  AUC_a1 : Constant  Value=40
  AUC_a2 : Constant  Value=O2CHMO
  G : Gain  Gain=O2CHMO
  Product : Product  RndMeth=Zero
  Sum1 : Sum  Inputs=-+|
  "if P02ART1>=80, AUC2 = 0 If PO2ART < 80, AUC2 = O2CHMO * (80-PO2ART);" : Switch  Threshold=80
  "if PO2ART>=40, AUC2 = AUC2 If PO2ART < 40, AUC2 = 40*O2CHMO" : Switch  Threshold=40
  AUC2 : Outport
  wires:
  "if P02ART1>=80, AUC2 = 0 If PO2ART < 80, AUC2 = O2CHMO * (80-PO2ART);"/1 -> "if PO2ART>=40, AUC2 = AUC2 If PO2ART < 40, AUC2 = 40*O2CHMO"/1  "AUC2"
  PO2ART/1 -> "if P02ART1>=80, AUC2 = 0 If PO2ART < 80, AUC2 = O2CHMO * (80-PO2ART);"/2, Sum1/1, "if PO2ART>=40, AUC2 = AUC2 If PO2ART < 40, AUC2 = 40*O2CHMO"/2
  "if PO2ART>=40, AUC2 = AUC2 If PO2ART < 40, AUC2 = 40*O2CHMO"/1 -> AUC2/1  "AUC2"
  G/1 -> "if P02ART1>=80, AUC2 = 0 If PO2ART < 80, AUC2 = O2CHMO * (80-PO2ART);"/3
  Sum1/1 -> G/1
  AUC1_a2/1 -> Sum1/2
  AUC_a/1 -> "if P02ART1>=80, AUC2 = 0 If PO2ART < 80, AUC2 = O2CHMO * (80-PO2ART);"/1
  AUC_a1/1 -> Product/2
  AUC_a2/1 -> Product/1
  Product/1 -> "if PO2ART>=40, AUC2 = AUC2 If PO2ART < 40, AUC2 = 40*O2CHMO"/3

== system myGuyton_corrected_new/Autonomic Control of the Circulation/AUC3, AUN, AUC6/AUN ==
  PA1 : Inport
  AUC1_a2 : Constant  Value=40
  AUC_a : Constant  Value=0
  Gin : Gain  Gain=0.04
  Gin1 : Gain  Gain=AUN1
  Sum1 : Sum  Inputs=-+|
  "if PA1>=40, AUN = 0 If PA1 < 40, AUN = 0.04 * (40-PA1);" : Switch  Threshold=40
  AUN : Outport
  wires:
  AUC_a/1 -> "if PA1>=40, AUN = 0 If PA1 < 40, AUN = 0.04 * (40-PA1);"/1
  AUC1_a2/1 -> Sum1/2
  Sum1/1 -> Gin/1
  Gin/1 -> "if PA1>=40, AUN = 0 If PA1 < 40, AUN = 0.04 * (40-PA1);"/3
  PA1/1 -> Sum1/1, "if PA1>=40, AUN = 0 If PA1 < 40, AUN = 0.04 * (40-PA1);"/2  "PA1"
  "if PA1>=40, AUN = 0 If PA1 < 40, AUN = 0.04 * (40-PA1);"/1 -> Gin1/1  "AUN"
  Gin1/1 -> AUN/1

== system myGuyton_corrected_new/Autonomic Control of the Circulation/AUC3, AUN, AUC6/Baroreceptors ==
  AU6A : Inport
  AUC1_a1 : Constant  Value=AU6_IC
  Gain2 : Gain  Gain=1/BAROTC
  Integrator : Integrator  InitialConditionSource=external
  Sum5 : Sum  Inputs=|+-
  AU6 : Outport
  wires:
  Sum5/1 -> Gain2/1
  Gain2/1 -> Integrator/1
  Integrator/1 -> Sum5/2, AU6/1  "AU6"
  AU6A/1 -> Sum5/1
  AUC1_a1/1 -> Integrator/2

== system myGuyton_corrected_new/Autonomic Control of the Circulation/Subsystem1/Subsystem3 ==
  AUTTL : Inport
  36 : Integrator  InitialConditionSource=external
  Constant3 : Constant  Value=AU1_IC
  Gain1 : Gain  Gain=1/AUDMP
  Sum2 : Sum  Inputs=|+-
  AU1 : Outport
  wires:
  Sum2/1 -> Gain1/1  "DAU"
  Gain1/1 -> 36/1
  Constant3/1 -> 36/2
  36/1 -> Sum2/2, AU1/1  "AU1"
  AUTTL/1 -> Sum2/1

== system myGuyton_corrected_new/Autoregulation/Muscle Local BF Control/Long-Term Muscle Auotoreg. ==
  In1 : Inport
  ARM10 : Gain  Gain=1/A4K2
  ARM11 : Integrator  InitialConditionSource=external
  IC_AMM2 : Constant  Value=AMM2_IC
  Sum4 : Sum  Inputs=|+-
  AMM2 : Outport
  wires:
  Sum4/1 -> ARM10/1
  ARM10/1 -> ARM11/1
  ARM11/1 -> Sum4/2, AMM2/1  "AMM2"
  In1/1 -> Sum4/1
  IC_AMM2/1 -> ARM11/2

== system myGuyton_corrected_new/Autoregulation/Muscle Local BF Control/Rapid Muscle Autoregulation ==
  POE : Inport
  ARM6 : Gain  Gain=1/A4K
  ARM7 : Integrator  InitialConditionSource=external
  IC_AMM1 : Constant  Value=AMM1_IC
  Sum2 : Sum  Inputs=|+-
  AMM1 : Outport
  wires:
  Sum2/1 -> ARM6/1
  ARM6/1 -> ARM7/1
  ARM7/1 -> Sum2/2, AMM1/1  "AMM1"
  POE/1 -> Sum2/1
  IC_AMM1/1 -> ARM7/2

== system myGuyton_corrected_new/Autoregulation/Non-Muscle Local BF Control/Intermediate Autoreg. ==
  POA : Inport
  ARN12 : Gain  Gain=1/A2K
  ARN13 : Integrator  InitialConditionSource=external
  IC_AR2 : Constant  Value=AR2_IC
  Sum5 : Sum  Inputs=|+-
  AR2 : Outport
  wires:
  ARN13/1 -> Sum5/2, AR2/1
  Sum5/1 -> ARN12/1
  ARN12/1 -> ARN13/1
  IC_AR2/1 -> ARN13/2
  POA/1 -> Sum5/1

== system myGuyton_corrected_new/Autoregulation/Non-Muscle Local BF Control/Long-Term Autoreg. ==
  POC : Inport
  ARN16 : Gain  Gain=1/A3K
  ARN17 : Integrator  InitialConditionSource=external
  IC_AR3 : Constant  Value=AR3_IC
  Sum4 : Sum  Inputs=|+-
  AR3 : Outport
  wires:
  ARN17/1 -> Sum4/2, AR3/1
  Sum4/1 -> ARN16/1
  ARN16/1 -> ARN17/1
  IC_AR3/1 -> ARN17/2
  POC/1 -> Sum4/1

== system myGuyton_corrected_new/Autoregulation/Non-Muscle Local BF Control/Rapid Autoreg. ==
  POB : Inport
  ARN6 : Gain  Gain=1/A1K
  ARN7 : Integrator  InitialConditionSource=external
  IC_AR1 : Constant  Value=AR1_IC
  Sum6 : Sum  Inputs=|+-
  AR1 : Outport
  wires:
  ARN7/1 -> Sum6/2, AR1/1
  Sum6/1 -> ARN6/1
  ARN6/1 -> ARN7/1
  IC_AR1/1 -> ARN7/2
  POB/1 -> Sum6/1

== system myGuyton_corrected_new/CIRCULATION/PAMK Calculation/PAMK DYNAMICS ==
  In1 : Inport
  Constant34 : Constant  Value=PAMK_IC
  Gain25 : Gain  Gain=1/KORTC
  Integrator5 : Integrator  InitialConditionSource=external
  Sum43 : Sum  Inputs=|+-
  PAMK : Outport
  wires:
  Sum43/1 -> Gain25/1
  Gain25/1 -> Integrator5/1
  Constant34/1 -> Integrator5/2
  Integrator5/1 -> Sum43/2, PAMK/1  "PAMK"
  In1/1 -> Sum43/1

== system myGuyton_corrected_new/CIRCULATION/QRN Calculation (FUN2)/FUN2 ==
  PRA1 : Inport  Orientation=left
  FUN2 : simulink/Lookup Tables/Lookup Table (n-D)  Orientation=left  numDimsPopupSelect=1  bp1=[-8, -6, -2, 4, 12]  bp2=[10,22,31]  bp3=[1:3]  bp4=[1:3]  bpcell={ [1:3], [1:3] }  explicitNumDims=2  searchMode=Binary Search  cacheBpFlag=off  vectorInputFlag=off  tableData=[0, 0.75, 2.6, 9.8, 13.5]  interpMethod=Cubic Spline  extrapMethod=None - Clip  rangeErrorMode=None
  QRN : Outport  Orientation=left
  wires:
  PRA1/1 -> FUN2/1
  FUN2/1 -> QRN/1  "QRN"

== system myGuyton_corrected_new/CIRCULATION/RMULT1 Calculation/Subsystem ==
  In1 : Inport
  Constant2 : Constant  Value=RMULT1_IC
  Gain25 : Gain  Gain=AUTOK
  Integrator : Integrator  InitialConditionSource=external
  Sum44 : Sum  Inputs=|+-
  Out1 : Outport
  wires:
  Sum44/1 -> Gain25/1
  Gain25/1 -> Integrator/1
  Integrator/1 -> Sum44/2, Out1/1  "RMULT1"
  Constant2/1 -> Integrator/2
  In1/1 -> Sum44/1

== system myGuyton_corrected_new/CIRCULATION/RV1 Calculation/DAMPING ==
  In1 : Inport  Orientation=left
  Constant1 : Constant  Orientation=left  Value=CN3_IC
  Gain5 : Gain  Orientation=left  Gain=1/30
  Integrator : Integrator  Orientation=left  InitialConditionSource=external
  Sum3 : Sum  Orientation=left  Inputs=|+-
  CN3 : Outport  Orientation=left
  wires:
  Sum3/1 -> Gain5/1
  Gain5/1 -> Integrator/1
  Constant1/1 -> Integrator/2
  Integrator/1 -> Sum3/2, CN3/1  "CN3"
  In1/1 -> Sum3/1

== system myGuyton_corrected_new/Capillary Dynamics, Tissue Fluid and Tissue Pprotein /VTS1 Calculation/VTS2 TF ==
  In1 : Inport
  Constant1 : Constant  Value=VTS2_IC
  Gain1 : Gain  Gain=TSSLTC
  Integrator : Integrator  InitialConditionSource=external
  Sum1 : Sum  Inputs=|+-
  VTS2 : Outport
  wires:
  Sum1/1 -> Gain1/1
  Gain1/1 -> Integrator/1
  Constant1/1 -> Integrator/2
  Integrator/1 -> Sum1/2, VTS2/1  "VTS2"
  In1/1 -> Sum1/1

== system myGuyton_corrected_new/KIDNEYS/GLPC Calculation/EFAFPR CALCULATION ==
  VP : Inport
  RFN : Inport  Port=2
  VB : Inport  Port=3
  GFN : Inport  Orientation=up  Port=4
  ANMARL6 : Saturate  UpperLimit=inf  LowerLimit=1
  Divide1 : Product  Inputs=*/  OutScaling=2^-10
  Divide8 : Product  Inputs=*/  OutScaling=2^-10
  Product : Product  RndMeth=Zero
  Sum1 : Sum  Inputs=|+-
  EFAFPR : Outport
  wires:
  Product/1 -> Divide1/1  "RFN*VP"
  VB/1 -> Divide1/2
  Divide1/1 -> Divide8/1, Sum1/1
  Sum1/1 -> Divide8/2
  Divide8/1 -> ANMARL6/1  "EFAFPR"
  RFN/1 -> Product/2
  GFN/1 -> Sum1/2
  VP/1 -> Product/1
  ANMARL6/1 -> EFAFPR/1  "EFAFPR"

== system myGuyton_corrected_new/KIDNEYS/GLPC Calculation/Subsystem ==
  In1 : Inport
  Constant1 : Constant  Value=GLPC_IC
  Gain1 : Gain  Gain=1/3
  Integrator : Integrator  InitialConditionSource=external
  Sum : Sum  Inputs=|+-
  Out1 : Outport
  wires:
  Sum/1 -> Gain1/1
  Gain1/1 -> Integrator/1
  Constant1/1 -> Integrator/2
  Integrator/1 -> Sum/2, Out1/1
  In1/1 -> Sum/1

== system myGuyton_corrected_new/KIDNEYS/PAR Calculation/PAR TF ==
  In1 : Inport
  Constant4 : Constant  Value=PAR_IC
  Gain1 : Gain  Gain=1/RCDFDP
  Integrator : Integrator  InitialConditionSource=external
  Sum3 : Sum  Inputs=|+-
  PAR : Outport
  wires:
  Sum3/1 -> Gain1/1
  Gain1/1 -> Integrator/1
  Constant4/1 -> Integrator/2
  Integrator/1 -> Sum3/2, PAR/1  "PAR"
  In1/1 -> Sum3/1

== system myGuyton_corrected_new/KIDNEYS/RFABD Calculation/DAMPING ==
  RFAB1 : Inport
  Constant5 : Constant  Value=RFAB_IC
  Gain5 : Gain  Gain=1/3
  Integrator : Integrator  InitialConditionSource=external
  Sum9 : Sum  Inputs=|+-
  RFAB : Outport
  wires:
  Sum9/1 -> Gain5/1
  Gain5/1 -> Integrator/1
  Constant5/1 -> Integrator/2
  Integrator/1 -> Sum9/2, RFAB/1  "RFAB"
  RFAB1/1 -> Sum9/1

== system myGuyton_corrected_new/KIDNEYS/RNAUG1 Calculation/Subsystem5 ==
  In1 : Inport  Orientation=left
  Constant8 : Constant  Orientation=left  Value=RNAUG1_IC
  Gain9 : Gain  Orientation=left  Gain=1/45
  Integrator : Integrator  Orientation=left  InitialConditionSource=external
  Sum10 : Sum  Orientation=left  Inputs=|+-
  RNAUG1 : Outport  Orientation=left
  wires:
  Sum10/1 -> Gain9/1
  Gain9/1 -> Integrator/1
  Constant8/1 -> Integrator/2
  Integrator/1 -> Sum10/2, RNAUG1/1
  In1/1 -> Sum10/1

== system myGuyton_corrected_new/Pulmonary Oxygen Uptake/O2VAD2 Calculation/O2VAD1 DYNAMICS ==
  In1 : Inport  Orientation=left
  Constant8 : Constant  Orientation=left  Value=O2VAD1_IC
  Gain4 : Gain  Orientation=left  Gain=0.0005
  Integrator : Integrator  Orientation=left  InitialConditionSource=external
  Sum7 : Sum  Orientation=left  Inputs=|+-
  O2VAD1 : Outport  Orientation=left
  wires:
  Gain4/1 -> Integrator/1  "DO2VAD"
  Sum7/1 -> Gain4/1
  Integrator/1 -> Sum7/2, O2VAD1/1
  Constant8/1 -> Integrator/2
  In1/1 -> Sum7/1
